simulink model "Ecotron"  (R2019b)
settings: Solver=FixedStepAuto  StartTime=0.0  StopTime=1  FixedStep=0.001  RelTol=1e-3  EnableMultiTasking=on
InitFcn:
  | EcoCoder_PreCheckLic();
libraries: CoderSF_BSW_Libs x228, SF_CanService_Libs x49, simulink x33, dspstat3 x6
(part 1 of 6)
settings Model: Param_HCUVersion=EH2275A02  Creator=btunc  LastModifiedBy=bayra
settings SolverCC: AutoInsertRateTranBlk=on
settings DataIOCC: SaveFormat=Structure  SignalLoggingSaveFormat=ModelDataLogs  SaveOutput=off  SignalLogging=off  DSMLogging=off  SaveTime=off  ReturnWorkspaceOutputs=off
settings OptimizationCC: DefaultParameterBehavior=Inlined  InlineInvariantSignals=on  EnhancedBackFolding=on  StrengthReduction=on  EnableMemcpy=off  PassReuseOutputArgsAs=Individual arguments  EfficientFloat2IntCast=on  LifeSpan=1  SimCompilerOptimization=on  OptimizeBlockOrder=speed  DifferentSizesBufferReuse=on  EfficientTunableParamExpr=on
settings DebuggingCC: AlgebraicLoopMsg=none  ArtificialAlgebraicLoopMsg=none  SaveWithDisabledLinksMsg=none  SaveWithParameterizedLinksMsg=none  CheckSSInitialOutputMsg=off  UnderspecifiedInitializationDetection=Classic  SignalResolutionControl=TryResolveAll  BlockPriorityViolationMsg=error  MinStepSizeMsg=none  InheritedTsInSrcMsg=none  MultiTaskDSMMsg=none  MultiTaskCondExecSysMsg=none  MultiTaskRateTransMsg=warning  TasksWithSamePriorityMsg=none  SigSpecEnsureSampleTimeMsg=none  IntegerOverflowMsg=error  Int32ToFloatConvMsg=none  ParameterPrecisionLossMsg=none  ParameterTunabilityLossMsg=none  FixptConstOverflowMsg=error  FcnCallInpInsideContextMsg=warning  UnconnectedInputMsg=error  UnconnectedOutputMsg=error  UnconnectedLineMsg=error  FrameProcessingCompatibilityMsg=none  BusObjectLabelMismatch=none  RootOutportRequireBusObject=none  UnknownTsInhSupMsg=none  ModelReferenceDataLoggingMessage=none  OperatingPointInterfaceChecksumMismatchMsg=none  SFUnusedDataAndEventsDiag=none  SFUnexpectedBacktrackingDiag=none  SFInvalidInputDataAccessInChartInitDiag=none  SFNoUnconditionalDefaultTransitionDiag=none  SFTransitionOutsideNaturalParentDiag=none  SFUnreachableExecutionPathDiag=none
settings HardwareCC: ProdBitPerPointer=32  ProdBitPerSizeT=32  ProdBitPerPtrDiffT=32  ProdLargestAtomicFloat=None  ProdWordSize=32  ProdHWDeviceType=Infineon->TriCore
settings ModelReferenceCC: UpdateModelReferenceTargets=Force  ModelReferenceNumInstancesAllowed=Single  PropagateSignalLabelsOutOfModel=off
settings SFSimCC: SFSimEcho=off  SimBuildMode=sf_make_clean  MATLABDynamicMemAlloc=off
settings RTWCC: Description=Ecotrons TC27x  SystemTargetFile=EcoCoderTC27x.tlc  GenerateMakefile=off  TemplateMakefile=ert_default_tmf  RTWVerbose=off  RetainRTWFile=on  RTWCompilerOptimization=on
settings CodeAppCC: IgnoreCustomStorageClasses=off  OperatorAnnotations=on  CustomSymbolStrGlobalVar=$N$M  CustomSymbolStrType=$N$M  CustomSymbolStrFcn=$N$M  CustomSymbolStrFcnArg=$N$M  CustomSymbolStrBlkIO=$N$M  CustomSymbolStrMacro=$N$M
settings STFCustomTargetCC: TargetLangStandard=C99 (ISO)  CodeReplacementLibrary=ANSI_C  UtilityFuncGeneration=Shared location  MultiwordLength=256  IncludeMdlTerminateFcn=off  CombineOutputUpdateFcns=on  SuppressErrorStatus=on  ERTCustomFileBanners=on  SupportNonFinite=off  SupportComplex=off  SupportContinuousTime=off  SupportNonInlinedSFcns=off  MATLABClassNameForMDSCustomization=Simulink.SoftwareTarget.ERTCustomization  SystemTargetFile=EcoCoderTC27x.tlc
settings ERTTargetCC: TargetLangStandard=C99 (ISO)  CodeReplacementLibrary=ANSI_C  UtilityFuncGeneration=Shared location  ParMdlRefBuildCompliant=off  CompOptLevelCompliant=off  ConcurrentExecutionCompliant=off  IncludeMdlTerminateFcn=off  SuppressErrorStatus=on  SupportNonFinite=off  SupportComplex=off  RemoveResetFunc=off  ModelStepFunctionPrototypeControlCompliant=off  CPPClassGenCompliant=off  UseToolchainInfoCompliant=off  GenerateASAP2=on  InlinedParameterPlacement=NonHierarchical  ERTCustomFileTemplate=MPC5644A_file_process.tlc  ERTFilePackagingFormat=Compact  PreserveIfCondition=on  ConvertIfToSwitch=off  PreserveExternInFcnDecls=off  SuppressUnreachableDefaultCases=off

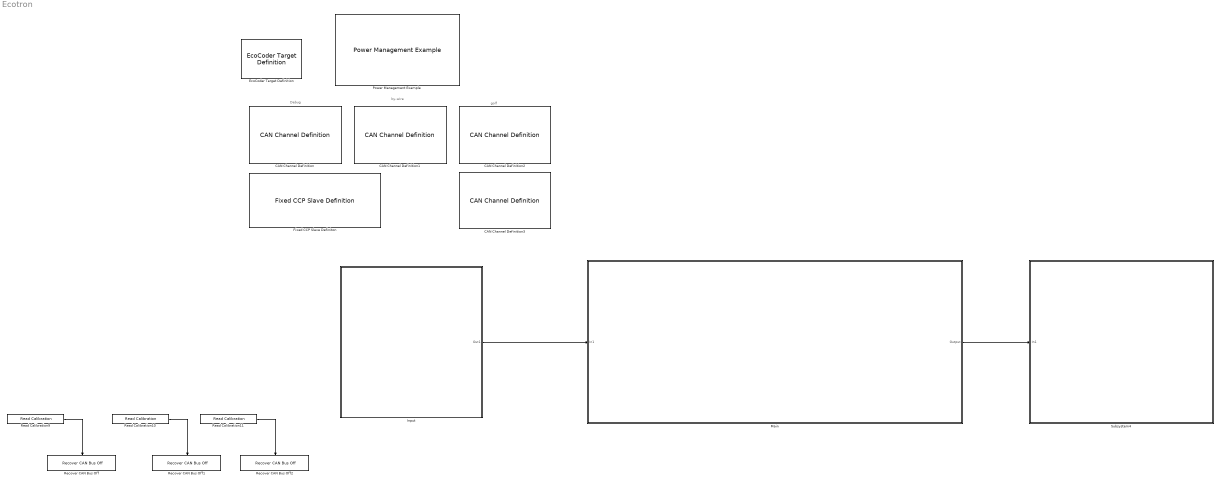
== system Ecotron ==
  note: golf
  note: by-wire
  note: Debug
  CAN Channel Definition : CoderSF_BSW_Libs/CAN/CAN Channel Definition  channel=CAN_A  can_en=on  can_idfilter=off  can_rxextended=off  can_rxMask=hex2dec('7ff')  can_rxID=hex2dec('100')  can_baudrateIndex=500  can_txbuffer_size=100  can_rxbuffer_size=1  can_en_fd=off  nominalSamplePoint=7500  can_baudrateIndex_data=500  fastSamplePoint=7500  canfd_txbuffer_size=5  EcoCoderBlockID=C001_CANDef
      settings: SourceProductName=EcoCoder Blocks
  CAN Channel Definition1 : CoderSF_BSW_Libs/CAN/CAN Channel Definition  channel=CAN_C  can_en=on  can_idfilter=off  can_rxextended=off  can_rxMask=hex2dec('7ff')  can_rxID=hex2dec('100')  can_baudrateIndex=500  can_txbuffer_size=20  can_rxbuffer_size=1  can_en_fd=off  nominalSamplePoint=7500  can_baudrateIndex_data=500  fastSamplePoint=7500  canfd_txbuffer_size=5  EcoCoderBlockID=C001_CANDef
      settings: SourceProductName=EcoCoder Blocks
  CAN Channel Definition2 : CoderSF_BSW_Libs/CAN/CAN Channel Definition  channel=CAN_B  can_en=on  can_idfilter=off  can_rxextended=off  can_rxMask=0  can_rxID=hex2dec('B5')  can_baudrateIndex=500  can_txbuffer_size=20  can_rxbuffer_size=1  can_en_fd=off  nominalSamplePoint=7500  can_baudrateIndex_data=500  fastSamplePoint=7500  canfd_txbuffer_size=5  EcoCoderBlockID=C001_CANDef
      settings: SourceProductName=EcoCoder Blocks
  CAN Channel Definition3 : CoderSF_BSW_Libs/CAN/CAN Channel Definition  channel=CAN_D  can_en=on  can_idfilter=off  can_rxextended=off  can_rxMask=hex2dec('7ff')  can_rxID=hex2dec('100')  can_baudrateIndex=500  can_txbuffer_size=20  can_rxbuffer_size=1  can_en_fd=off  nominalSamplePoint=7500  can_baudrateIndex_data=500  fastSamplePoint=7500  canfd_txbuffer_size=5  EcoCoderBlockID=C001_CANDef
      settings: SourceProductName=EcoCoder Blocks
  EcoCoder Target Definition : CoderSF_BSW_Libs/EcoCoder Target Definition  targetECU=EH2275A02  EcoCoderBlockID=T001_Target  enNoTriggerCall=on  flgBlockReduction=on  flgShowDebugDisp=off  flgDisTargetOutFIleCounter=off  flgClearAllOldFiles=on  tc275_cal_len=hex2dec('00008000')  ipVal='192.168.0.123'  userName='nvidia'  passWord='nvidia'  workSpace='~/cmake_ws'  libraryLink=''  enExt=on  portExt=17725  internal_flash=[hex2dec('00020000'),hex2dec('000E0000')]  cal_rom_phy=[hex2dec('00010000'),hex2dec('00002000')]  cal_ram_wp=[hex2dec('4000F000'),hex2dec('00002000')]  cal_ram_msm=[hex2dec('40000000'),hex2dec('00002000')]  var_ram_wp=[hex2dec('40002000'),hex2dec('0000D000')]  write_back_fixed_ram=[hex2dec('40011000'),hex2dec('00001000')]  write_back_unfixed_ram=[hex2dec('40012000'),hex2dec('00001000')]  stack=[hex2dec('40013000'),hex2dec('00001000')]
      settings: AttributesFormatString=Target :%<targetECU>  SourceProductName=EcoCoder Blocks
  Fixed CCP Slave Definiton : CoderSF_BSW_Libs/CCP/Fixed CCP Slave Definition  ccp_enSet=on  ccp_disASW=on  channel=CAN_A  stationaddressSet=hex2dec('0112')  croidSet=hex2dec('100')  dtoidSet=hex2dec('101')  daqidSet=[hex2dec('101') hex2dec('101') hex2dec('101') hex2dec('102')]  daqpidSet=[hex2dec('0') hex2dec('3C') hex2dec('78') hex2dec('0')]  daqlenSet=[hex2dec('0') hex2dec('20') hex2dec('30') hex2dec('30')]  daqperSet=[5 20 100 0]  EcoCoderBlockID=C002_CCP21Conf
      settings: SourceProductName=EcoCoder Blocks
  Input : Subsystem
  "Main " : Subsystem
  Power Management Example : CoderSF_BSW_Libs/System Management Blocks/Power Management Example  Priority=1  flgKeyFromIn=off  tasktimeIndex=Task_L5ms  tKeyOffDelaySet=0.5  flgResetSWEnSet=1  tDbncKeyOffFallSet=0.1  tDbncKeyOffRiseSet=0.1  facAd2VoltSet=109/27846  uKeyOffThrSet=1  uKeyOnHystSet=1  flgCANRxLiveCheckEn=0  flgEnPwrDwnFailReset=0  flgNVMEn=off  tShtDwnWait=500  flgPwrDwnByEdgeTrigger=off  EcoCoderBlockID=PME001_Def
      settings: AttributesFormatString=Priority:%<Priority>  SourceProductName=EcoCoder Blocks
  Read Calibration10 : CoderSF_BSW_Libs/Calibration & Measurement/Read Calibration  variable_name=CANB_recover  variable_value=0  variable_type=single  variable_min=[]  variable_max=[]  unitStr=""  descStr=""
      settings: AttributesFormatString=value:%<variable_value> type:%<variable_type> max:%<variable_max> Min:%<variable_min>  SourceProductName=EcoCoder Blocks
  Read Calibration11 : CoderSF_BSW_Libs/Calibration & Measurement/Read Calibration  variable_name=CANC_recover  variable_value=0  variable_type=single  variable_min=[]  variable_max=[]  unitStr=""  descStr=""
      settings: AttributesFormatString=value:%<variable_value> type:%<variable_type> max:%<variable_max> Min:%<variable_min>  SourceProductName=EcoCoder Blocks
  Read Calibration9 : CoderSF_BSW_Libs/Calibration & Measurement/Read Calibration  variable_name=CANA_recover  variable_value=0  variable_type=single  variable_min=[]  variable_max=[]  unitStr=""  descStr=""
      settings: AttributesFormatString=value:%<variable_value> type:%<variable_type> max:%<variable_max> Min:%<variable_min>  SourceProductName=EcoCoder Blocks
  Recover CAN Bus Off : CoderSF_BSW_Libs/CAN/Recover CAN Bus Off  channel=CAN_A
      settings: SourceProductName=EcoCoder Blocks
  Recover CAN Bus Off1 : CoderSF_BSW_Libs/CAN/Recover CAN Bus Off  channel=CAN_B
      settings: SourceProductName=EcoCoder Blocks
  Recover CAN Bus Off2 : CoderSF_BSW_Libs/CAN/Recover CAN Bus Off  channel=CAN_C
      settings: SourceProductName=EcoCoder Blocks
  Subsystem4 : Subsystem
  wires:
  Read Calibration9/1 -> Recover CAN Bus Off/Enable
  Read Calibration10/1 -> Recover CAN Bus Off1/Enable
  Read Calibration11/1 -> Recover CAN Bus Off2/Enable
  Input/1(Out1) -> "Main "/1(In1)
  "Main "/1(Output) -> Subsystem4/1(In1)

== system Ecotron/Input ==
  Bus Creator : BusCreator  Inputs=3
  By-wire : Subsystem
  Golf : Subsystem
  PC : Subsystem
  Out1 : Outport
  wires:
  By-wire/1(bywire) -> Bus Creator/1  "By-wire"
  Golf/1("Golf ") -> Bus Creator/2  "vehicle"
  Bus Creator/1 -> Out1/1
  PC/1(Output) -> Bus Creator/3  "PC"

== system Ecotron/Main  ==
  In1 : Inport
  Bus Creator : BusCreator  Inputs=2
  Bus Creator1 : BusCreator  Inputs=3
  Bus Creator2 : BusCreator  Inputs=5
  Err Handler : Subsystem
  Gear : Subsystem
  LateralControl : Subsystem
  "LongControl " : Subsystem
  Mode Select : Subsystem
  PDS StartupShutdown : Subsystem
  Output : Outport
  wires:
  In1/1 -> Bus Creator1/1, Bus Creator/1, Err Handler/1(In1)  "input"
  Err Handler/1(Out1) -> Bus Creator/2, Bus Creator1/3  "Errors"
  Bus Creator/1 -> Mode Select/1(In1)
  Mode Select/1(Output) -> Bus Creator1/2  "mode"
  Bus Creator1/1 -> Bus Creator2/1, LateralControl/1(In1), PDS StartupShutdown/1(In1), "LongControl "/1(In1), Gear/1(input)  "input"
  Gear/1(Output) -> Bus Creator2/2  "gearMSGTrigger"
  "LongControl "/1(Out1) -> Gear/2(longitudinal), Bus Creator2/3  "longitudinal"
  Bus Creator2/1 -> Output/1
  LateralControl/1(Out1) -> Bus Creator2/4  "Steer"
  PDS StartupShutdown/1(Out1) -> Bus Creator2/5  "PDSscript"

== system Ecotron/Subsystem4 ==
  In1 : Inport
  Brake : Subsystem
  Bus Selector : BusSelector  OutputSignals=Steer,gearMSGTrigger
  "Button cntrl " : Subsystem
  Gas : Subsystem
  Gear : Subsystem
  PC : Subsystem
  PDS : Subsystem
  "Steering Control " : Subsystem
  wires:
  Bus Selector/2 -> Gear/1(Gear_trigger)  "<gearMSGTrigger>"
  Bus Selector/1 -> "Steering Control "/1(inputBus)  "<Steer>"
  In1/1 -> Brake/1(Input), Gas/1(input), PC/1(In1), "Button cntrl "/1(Input), PDS/1(In1), Bus Selector/1

== system Ecotron/Input/By-wire ==
  Bus Creator : BusCreator  Inputs=4
  PDS : Subsystem
  Robeff Brake ECU : Subsystem
  Robeff EPAS ECU : Subsystem
  Throttle Controller : Subsystem
  bywire : Outport
  wires:
  Robeff EPAS ECU/1(EPAS) -> Bus Creator/1  "EPAS"
  Throttle Controller/1(Throttle) -> Bus Creator/3  "Throttle"
  Bus Creator/1 -> bywire/1
  PDS/1(PDS) -> Bus Creator/4  "PDS"
  Robeff Brake ECU/1(RBF_Brake) -> Bus Creator/2  "RBF_Brake"

== system Ecotron/Input/Golf ==
  BCM_01 : Subsystem
  Brake : Subsystem
  Brake and Steering Feedback Echo : Subsystem
  Bus Creator : BusCreator  Inputs=16
  EPB_01 : Subsystem
  ESP_05 : Subsystem
  Gateway_72 : Subsystem
  Getriebe_1 : Subsystem
  Getriebe_11 : Subsystem
  Getriebe_2 : Subsystem
  Kombi_02 : Subsystem
  LWl : Subsystem
  Motor_11 : Subsystem
  Motor_12 : Subsystem
  Motor_14 : Subsystem
  Motor_20 : Subsystem
  Subsystem : Subsystem
  WheelSpeed : Subsystem
  "Golf " : Outport
  wires:
  WheelSpeed/1("WheelSpeed ") -> Bus Creator/3  "WheelSpeed"
  Brake/1(Brake) -> Bus Creator/2  "BrakePedal"
  LWl/1(LWI) -> Bus Creator/1  "LWI"
  Bus Creator/1 -> "Golf "/1
  EPB_01/1(Acceleration) -> Bus Creator/6  "Acceleration"
  Motor_20/1(Accelerator_Pedal) -> Bus Creator/7  "Acc_Pedal_POS"
  Motor_14/1(KL75) -> Bus Creator/8  "Kontak"
  Gateway_72/1(Signal) -> Bus Creator/9  "Signal"
  Motor_12/1(MatorRPM) -> Bus Creator/5  "MotorRotationSpeed"
  Subsystem/1(GearSwitch) -> Bus Creator/4  "gear"
  BCM_01/1(HazardLight) -> Bus Creator/10  "Hazard"
  Kombi_02/1(Fuel_Tank) -> Bus Creator/11  "Fuel"
  Motor_11/1(MatorTorque) -> Bus Creator/12  "MotorTorque"
  Getriebe_11/1(GearLevel) -> Bus Creator/13  "GearLevel"
  Getriebe_1/1(ACC) -> Bus Creator/14  "ACC"
  Getriebe_2/1(TSK) -> Bus Creator/15  "TSK"
  ESP_05/1(ESP_05) -> Bus Creator/16  "BrakePressure"

== system Ecotron/Input/PC ==
  Bus Creator : BusCreator  Inputs=4
  FrontWheelCommands : Subsystem
  LongitudinalCommands : Subsystem
  LongitudinalCommandsV2 : Subsystem
  Vehicle_Commands : Subsystem
  Output : Outport
  wires:
  Vehicle_Commands/1(Out1) -> Bus Creator/1  "VehicleCMD"
  FrontWheelCommands/1(Out2) -> Bus Creator/2  "FrontWheelCMD"
  LongitudinalCommands/1(Out2) -> Bus Creator/3  "LongCMD"
  LongitudinalCommandsV2/1(Out2) -> Bus Creator/4  "LongV2CMD"
  Bus Creator/1 -> Output/1

== system Ecotron/Main /Err Handler ==
  In1 : Inport
  Bus Creator : BusCreator  Inputs=6
  Check Brake Err : Subsystem
  Check EPAS Err : Subsystem
  Check PDS Errors : Subsystem
  Check Throttle ECU Errors : Subsystem
  MotorStatus : Subsystem
  Subsystem : Subsystem
  Out1 : Outport
  wires:
  Check Brake Err/1(Out1) -> Bus Creator/5  "Brake_Err"
  In1/1 -> Subsystem/1(In1), Check Brake Err/1(In1), Check EPAS Err/1(In1), MotorStatus/1(In1), Check PDS Errors/1(In1), Check Throttle ECU Errors/1(In1)
  MotorStatus/1(Motor) -> Bus Creator/1  "Motor"
  Check PDS Errors/1(Out1) -> Bus Creator/2  "PDS_Err"
  Check Throttle ECU Errors/1(Out1) -> Bus Creator/3  "Throttle_ECU_Err"
  Bus Creator/1 -> Out1/1
  Check EPAS Err/1(Epas_Errors) -> Bus Creator/4  "Epas_Err"
  Subsystem/1(Out1) -> Bus Creator/6  "PC_HeartBeatErr"

== system Ecotron/Main /Gear ==
  input : Inport
  longitudinal : Inport  Port=2
  " Override Probe" : CoderSF_BSW_Libs/Calibration & Measurement/ Override Probe  variableName=Set_GearEnable  variableValue=1  overrideValue=0  variableDataType=single  variableMin=[]  variableMax=[]  variableUnitStr=""  variableDescStr=""
      settings: SourceProductName=EcoCoder Blocks
  Bus Selector : BusSelector  OutputSignals=input.vehicle.gear.GOLF_CurrentGear,input.vehicle.gear.Msg.Available,input.vehicle.Acceleration.GOLF_HandBrakeStatus,input.PC.VehicleCMD.PC_gear,mode
  Bus Selector1 : BusSelector  OutputSignals=stopMode
  Compare To Constant : simulink/Logic and Bit Operations/Compare To Constant  relop===  const=1  OutDataTypeStr=boolean
  Constant : Constant  OutDataTypeStr=uint8
  Gear_Control : Subsystem
  Switch : Switch  Criteria=u2 > Threshold  Threshold=0.5
  Output : Outport
  wires:
  Bus Selector/2 -> Gear_Control/2(Available)  "<Available>"
  Bus Selector/1 -> Gear_Control/1(GOLF_CurrentGear)  "<GOLF_CurrentGear>"
  input/1 -> Bus Selector/1
  " Override Probe"/1 -> Gear_Control/4(Enable)  "Set_GearEnableOvrMsr"
  Gear_Control/1(Gear_Trigger) -> Output/1
  Bus Selector/3 -> Switch/2  "<GOLF_HandBrakeStatus>"
  Constant/1 -> Switch/1
  Switch/1 -> Gear_Control/3("Set_gear ")
  Bus Selector/4 -> Switch/3  "<PC_gear>"
  Bus Selector/5 -> " Override Probe"/1  "<mode>"
  longitudinal/1 -> Bus Selector1/1
  Bus Selector1/1 -> Compare To Constant/1  "<stopMode>"
  Compare To Constant/1 -> Gear_Control/5(ParkEnable)

== system Ecotron/Main /LateralControl ==
  In1 : Inport
  Bus Creator : BusCreator  Inputs=4
  Bus Selector : BusSelector  OutputSignals=mode,input.vehicle.WheelSpeed.GOLF_BRWheelSpeed,input.By-wire.EPAS.EPAS_Msg3.EPAS_DriverIntervention_overrideOvrMsr,input.PC.FrontWheelCMD.PC_SetFrontWheelAngle
  Chart : Stateflow chart  BlockKeywords=__PRM__SERIALIZED__DATA__:Stateflow Chart,Stateflow Diagram  TreatAsAtomicUnit=on
  Read Calibration : CoderSF_BSW_Libs/Calibration & Measurement/Read Calibration  variable_name=EPAS_MaxSpeed  variable_value=360  variable_type=single  variable_min=[]  variable_max=[]  unitStr=""  descStr=""
      settings: AttributesFormatString=value:%<variable_value> type:%<variable_type> max:%<variable_max> Min:%<variable_min>  SourceProductName=EcoCoder Blocks
  Steering Map : Subsystem
  Write and Read Measurement : CoderSF_BSW_Libs/Calibration & Measurement/Write and Read Measurement  variable_name=debug_EPASmode  variable_value=0  variable_type=uint8  numD=1  unitStr=""  descStr=""
      settings: AttributesFormatString=type:%<variable_type> Dimensions:%<numD>  SourceProductName=EcoCoder Blocks
  Write and Read Measurement1 : CoderSF_BSW_Libs/Calibration & Measurement/Write and Read Measurement  variable_name=debug_EPASsetsteer  variable_value=0  variable_type=single  numD=1  unitStr=""  descStr=""
      settings: AttributesFormatString=type:%<variable_type> Dimensions:%<numD>  SourceProductName=EcoCoder Blocks
  Write and Read Measurement2 : CoderSF_BSW_Libs/Calibration & Measurement/Write and Read Measurement  variable_name=debug_EPASspeedlimit  variable_value=0  variable_type=single  numD=1  unitStr=""  descStr=""
      settings: AttributesFormatString=type:%<variable_type> Dimensions:%<numD>  SourceProductName=EcoCoder Blocks
  Write and Read Measurement3 : CoderSF_BSW_Libs/Calibration & Measurement/Write and Read Measurement  variable_name=debug_EPAS_ECU_reset  variable_value=0  variable_type=boolean  numD=1  unitStr=""  descStr=""
      settings: AttributesFormatString=type:%<variable_type> Dimensions:%<numD>  SourceProductName=EcoCoder Blocks
  Out1 : Outport
  wires:
  In1/1 -> Bus Selector/1
  Bus Selector/1 -> Chart/1(AutonomyEnable)  "<mode>"
  Bus Creator/1 -> Out1/1
  Write and Read Measurement/1 -> Bus Creator/1  "debug_EPASmode"
  Write and Read Measurement1/1 -> Bus Creator/2  "debug_EPASsetsteer"
  Write and Read Measurement2/1 -> Bus Creator/3  "debug_EPASspeedlimit"
  Chart/1(EPAS_mode) -> Write and Read Measurement/1
  Chart/2(EPAS_SteeringPosCMD) -> Write and Read Measurement1/1
  Chart/3(EPAS_Speedlimit) -> Write and Read Measurement2/1
  Chart/4(Epas_ECU_reset) -> Write and Read Measurement3/1
  Write and Read Measurement3/1 -> Bus Creator/4  "debug_EPAS_ECU_reset"
  Bus Selector/4 -> Steering Map/1(Wheel Rad)  "<PC_SetFrontWheelAngle>"
  Read Calibration/1 -> Chart/4(MaxEPASSpeed)
  Bus Selector/2 -> Chart/2(Vehicle_Speed)  "<GOLF_BRWheelSpeed>"
  Bus Selector/3 -> Chart/3(EPAS_intervention)  "<EPAS_DriverIntervention_overrideOvrMsr>"
  Steering Map/1(Steering Wheel Degree) -> Chart/5(Set_SteeringPos)

== system Ecotron/Main /LongControl  ==
  In1 : Inport
  ACC Control : Subsystem
  Brake Calib logic : Subsystem
  Bus Creator : BusCreator  Inputs=4
  Bus Selector : BusSelector  OutputSignals=mode,input.PC.VehicleCMD.PC_LongMode,input.PC.LongV2CMD.PC_SetBrakePos,input.PC.LongV2CMD.PC_SetGasPos
  Chart : Stateflow chart  Commented=on  BlockKeywords=__PRM__SERIALIZED__DATA__:Stateflow Chart,Stateflow Diagram  TreatAsAtomicUnit=on
  Out1 : Outport
  wires:
  Bus Selector/1 -> Chart/1(AutonomyEnable)  "<mode>"
  Bus Selector/2 -> Chart/2(LongMode)  "<PC_LongMode>"
  Bus Selector/3 -> Chart/3(PC_Brake)  "<PC_SetBrakePos>"
  Bus Selector/4 -> Chart/4(PC_Throttle)  "<PC_SetGasPos>"
  Bus Creator/1 -> Out1/1
  In1/1 -> Brake Calib logic/1(In1), ACC Control/1(In2), Bus Selector/1
  Brake Calib logic/1(Out1) -> Bus Creator/3  "BrakeCalibCMD"
  ACC Control/1(gas) -> Bus Creator/2  "Throttle_out"
  ACC Control/2(brake) -> Bus Creator/1  "Brake_out"
  ACC Control/3(StopMode) -> Bus Creator/4  "stopMode"

== system Ecotron/Main /Mode Select ==
  In1 : Inport
  " Override Probe" : CoderSF_BSW_Libs/Calibration & Measurement/ Override Probe  variableName=debug_otonomEnable  variableValue=0  overrideValue=0  variableDataType=boolean  variableMin=[]  variableMax=[]  variableUnitStr=""  variableDescStr=""
      settings: SourceProductName=EcoCoder Blocks
  " Override Probe1" : CoderSF_BSW_Libs/Calibration & Measurement/ Override Probe  variableName=debug_otonomDisable  variableValue=0  overrideValue=0  variableDataType=boolean  variableMin=[]  variableMax=[]  variableUnitStr=""  variableDescStr=""
      settings: SourceProductName=EcoCoder Blocks
  " Override Probe2" : CoderSF_BSW_Libs/Calibration & Measurement/ Override Probe  variableName=debug_PCheardbeat  variableValue=0  overrideValue=0  variableDataType=boolean  variableMin=[]  variableMax=[]  variableUnitStr=""  variableDescStr=""
      settings: SourceProductName=EcoCoder Blocks
  Bus Selector1 : BusSelector  OutputSignals=Errors.Motor.isMotorRunning,Errors.Motor.Kl75,Errors.PDS_Err.PDS_HeartbeatErr,Errors.PDS_Err.PDS_BUSErr,Errors.PDS_Err.By-wirePowerErr,Errors.PDS_Err.EPASPowerErr,Errors.PDS_Err.BrakePowerErr,Errors.Throttle_ECU_Err.GasPedalintervention,Errors.Epas_Err.EPAS_SystemErr,Errors.Brake_Err.Brake_SystemErr,input.By-wire.EPAS.EPAS_Msg3.EPAS_DriverIntervention_overrideOvrMsr,input.By-wire.RBF_Brake.EPAS_Msg3.BBW_DriverIntervention,Errors.Brake_Err.Brake_HeartBeatErr,Errors.Epas_Err.EPAS_HeartbeatErr,Errors.PC_HeartBeatErr
  Bus Selector2 : BusSelector  OutputSignals=input.PC.VehicleCMD.PC_mode,input.vehicle.Acceleration.GOLF_HandBrakeStatus
  Chart : Stateflow chart  BlockKeywords=__PRM__SERIALIZED__DATA__:Stateflow Chart,Stateflow Diagram  TreatAsAtomicUnit=on
  Compare To Constant : simulink/Logic and Bit Operations/Compare To Constant  relop===  const=1  OutDataTypeStr=boolean
  Compare To Constant1 : simulink/Logic and Bit Operations/Compare To Constant  relop=~=  const=1  OutDataTypeStr=boolean
  NOT : Logic  Operator=NOT  IconShape=distinctive  AllPortsSameDT=off  OutDataTypeStr=boolean
  NOT1 : Logic  Operator=NOT  IconShape=distinctive  AllPortsSameDT=off  OutDataTypeStr=boolean
  OR : Logic  Operator=OR  Inputs=15  IconShape=distinctive  AllPortsSameDT=off  OutDataTypeStr=boolean
  Rising Edge1 : CoderSF_BSW_Libs/Application Base Blocks/Rising Edge  InitialCondition=off
      settings: SourceProductName=EcoCoder Blocks
  Rising Edge2 : CoderSF_BSW_Libs/Application Base Blocks/Rising Edge  InitialCondition=off
      settings: SourceProductName=EcoCoder Blocks
  Rising Edge3 : CoderSF_BSW_Libs/Application Base Blocks/Rising Edge  InitialCondition=off
      settings: SourceProductName=EcoCoder Blocks
  Write Measurement : CoderSF_BSW_Libs/Calibration & Measurement/Write Measurement  variable_name=debug_Mode  variable_value=0  variable_type=boolean  numD=1  unitStr=""  descStr=""
      settings: AttributesFormatString=type:%<variable_type> Dimensions:%<numD>  SourceProductName=EcoCoder Blocks
  Write Measurement3 : CoderSF_BSW_Libs/Calibration & Measurement/Write Measurement  variable_name=debug_Errors  variable_value=0  variable_type=boolean  numD=1  unitStr=""  descStr=""
      settings: AttributesFormatString=type:%<variable_type> Dimensions:%<numD>  SourceProductName=EcoCoder Blocks
  Output : Outport
  wires:
  In1/1 -> Bus Selector1/1, Bus Selector2/1
  Bus Selector1/1 -> NOT/1  "<isMotorRunning>"
  Bus Selector1/2 -> NOT1/1  "<Kl75>"
  Bus Selector1/3 -> OR/3  "<PDS_HeartbeatErr>"
  Bus Selector1/4 -> OR/4  "<PDS_BUSErr>"
  Bus Selector1/5 -> OR/5  "<By-wirePowerErr>"
  Bus Selector1/6 -> OR/6  "<EPASPowerErr>"
  Bus Selector1/7 -> OR/7  "<BrakePowerErr>"
  Bus Selector1/8 -> OR/8  "<GasPedalintervention>"
  Bus Selector1/9 -> OR/9  "<EPAS_SystemErr>"
  Bus Selector1/10 -> OR/10  "<Brake_SystemErr>"
  OR/1 -> Chart/1(Errors), Write Measurement3/1
  " Override Probe"/1 -> Chart/2(AutonomyEnable)  "debug_otonomEnableOvrMsr"
  Chart/1(Mode) -> Output/1, Write Measurement/1  "autonomy_Enable"
  NOT/1 -> OR/1
  NOT1/1 -> OR/2
  Bus Selector1/11 -> Rising Edge2/1  "<EPAS_DriverIntervention_overrideOvrMsr>"
  Bus Selector1/12 -> Rising Edge1/1  "<BBW_DriverIntervention>"
  Bus Selector1/13 -> OR/13  "<Brake_HeartBeatErr>"
  Bus Selector1/14 -> OR/14  "<EPAS_HeartbeatErr>"
  Bus Selector2/1 -> Compare To Constant1/1, Compare To Constant/1  "<PC_mode>"
  Rising Edge1/1 -> OR/12
  Rising Edge2/1 -> OR/11
  Compare To Constant/1 -> Rising Edge3/1
  Bus Selector1/15 -> " Override Probe2"/1  "<PC_HeartBeatErr>"
  Rising Edge3/1 -> " Override Probe"/1
  Compare To Constant1/1 -> " Override Probe1"/1
  " Override Probe1"/1 -> Chart/3(AutonomyDisable)  "debug_otonomDisableOvrMsr"
  Bus Selector2/2 -> Chart/4(HandBrake)  "<GOLF_HandBrakeStatus>"
  " Override Probe2"/1 -> OR/15  "debug_PCheardbeatOvrMsr"

== system Ecotron/Main /PDS StartupShutdown ==
  In1 : Inport
  Bus Creator : BusCreator  Inputs=3
  Bus Selector : BusSelector  OutputSignals=input.By-wire.PDS.Status.PDS_Status1
  Chart : Stateflow chart  BlockKeywords=__PRM__SERIALIZED__DATA__:Stateflow Chart,Stateflow Diagram  TreatAsAtomicUnit=on
  Compare To Constant : simulink/Logic and Bit Operations/Compare To Constant  relop=>  const=0  OutDataTypeStr=boolean
  Falling Edge : CoderSF_BSW_Libs/Application Base Blocks/Falling Edge  InitialCondition=off
      settings: SourceProductName=EcoCoder Blocks
  Rising Edge : CoderSF_BSW_Libs/Application Base Blocks/Rising Edge  InitialCondition=on
      settings: SourceProductName=EcoCoder Blocks
  Out1 : Outport
  wires:
  In1/1 -> Bus Selector/1
  Bus Selector/1 -> Compare To Constant/1  "<PDS_Status1>"
  Compare To Constant/1 -> Falling Edge/1, Rising Edge/1
  Rising Edge/1 -> Chart/1(risingedge)
  Falling Edge/1 -> Chart/2(fallingedge)
  Chart/1(Channel) -> Bus Creator/1
  Chart/2(Onoff) -> Bus Creator/2
  Chart/3(Msgtrigger) -> Bus Creator/3
  Bus Creator/1 -> Out1/1

== system Ecotron/Subsystem4/Brake ==
  Input : Inport
  " Override Probe" : CoderSF_BSW_Libs/Calibration & Measurement/ Override Probe  variableName=Set_Brake_Pos  variableValue=0  overrideValue=0  variableDataType=single  variableMin=[]  variableMax=[]  variableUnitStr=""  variableDescStr=""
      settings: SourceProductName=EcoCoder Blocks
  " Override Probe1" : CoderSF_BSW_Libs/Calibration & Measurement/ Override Probe  variableName=Brake_Reset  variableValue=0  overrideValue=0  variableDataType=uint8  variableMin=[]  variableMax=[]  variableUnitStr=""  variableDescStr=""
      settings: SourceProductName=EcoCoder Blocks
  Bus Selector : BusSelector  OutputSignals=longitudinal.Brake_out,input.mode,Steer.debug_EPAS_ECU_reset,longitudinal.BrakeCalibCMD
  Constant6 : Constant  Value=0
  Read Calibration1 : CoderSF_BSW_Libs/Calibration & Measurement/Read Calibration  variable_name=Brake_ControlMode  variable_value=0  variable_type=single  variable_min=[]  variable_max=[]  unitStr=""  descStr=""
      settings: AttributesFormatString=value:%<variable_value> type:%<variable_type> max:%<variable_max> Min:%<variable_min>  SourceProductName=EcoCoder Blocks
  Read Calibration19 : CoderSF_BSW_Libs/Calibration & Measurement/Read Calibration  variable_name=Brake_SetDuty  variable_value=0  variable_type=uint8  variable_min=[]  variable_max=[]  unitStr=""  descStr=""
      settings: AttributesFormatString=value:%<variable_value> type:%<variable_type> max:%<variable_max> Min:%<variable_min>  SourceProductName=EcoCoder Blocks
  Send CAN Message 2 : SF_CanService_Libs/Send CAN Message   typeCAN=Connected  channel=CAN_C  mEn=off  msgInfo=RBF_DBW40_brake  msgItermStore=CommandMessage  msgIterm=CommandMessage  motoBit=off  flgNoFixed=on  tSample=Task_L10ms  modeCode=Parameterless  modeRound=Zero
  Switch2 : Switch  Criteria=u2 > Threshold  OutDataTypeStr=single
  wires:
  Read Calibration19/1 -> Send CAN Message 2/2
  " Override Probe1"/1 -> Send CAN Message 2/4  "Brake_ResetOvrMsr"
  " Override Probe"/1 -> Send CAN Message 2/3  "Set_Brake_PosOvrMsr"
  Input/1 -> Bus Selector/1
  Constant6/1 -> Switch2/3
  Switch2/1 -> " Override Probe"/1
  Bus Selector/2 -> Switch2/2  "<mode>"
  Bus Selector/1 -> Switch2/1  "<Brake_out>"
  Read Calibration1/1 -> Send CAN Message 2/1  "Brake_ControlModeOvrMsr"
  Bus Selector/3 -> " Override Probe1"/1  "<debug_EPAS_ECU_reset>"
  Bus Selector/4 -> Send CAN Message 2/5  "<BrakeCalibCMD>"

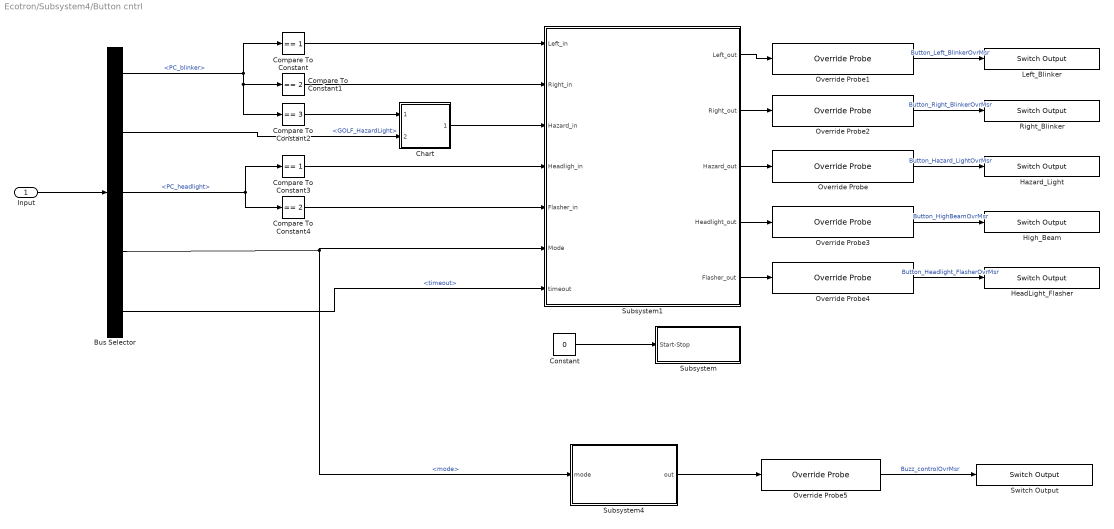
== system Ecotron/Subsystem4/Button cntrl  ==
  Input : Inport
  " Override Probe" : CoderSF_BSW_Libs/Calibration & Measurement/ Override Probe  variableName=Button_Hazard_Light  variableValue=0  overrideValue=0  variableDataType=boolean  variableMin=[]  variableMax=[]  variableUnitStr=""  variableDescStr=""
      settings: SourceProductName=EcoCoder Blocks
  " Override Probe1" : CoderSF_BSW_Libs/Calibration & Measurement/ Override Probe  variableName=Button_Left_Blinker  variableValue=0  overrideValue=0  variableDataType=boolean  variableMin=[]  variableMax=[]  variableUnitStr=""  variableDescStr=""
      settings: SourceProductName=EcoCoder Blocks
  " Override Probe2" : CoderSF_BSW_Libs/Calibration & Measurement/ Override Probe  variableName=Button_Right_Blinker  variableValue=0  overrideValue=0  variableDataType=boolean  variableMin=[]  variableMax=[]  variableUnitStr=""  variableDescStr=""
      settings: SourceProductName=EcoCoder Blocks
  " Override Probe3" : CoderSF_BSW_Libs/Calibration & Measurement/ Override Probe  variableName=Button_HighBeam  variableValue=0  overrideValue=0  variableDataType=boolean  variableMin=[]  variableMax=[]  variableUnitStr=""  variableDescStr=""
      settings: SourceProductName=EcoCoder Blocks
  " Override Probe4" : CoderSF_BSW_Libs/Calibration & Measurement/ Override Probe  variableName=Button_Headlight_Flasher  variableValue=0  overrideValue=0  variableDataType=boolean  variableMin=[]  variableMax=[]  variableUnitStr=""  variableDescStr=""
      settings: SourceProductName=EcoCoder Blocks
  " Override Probe5" : CoderSF_BSW_Libs/Calibration & Measurement/ Override Probe  variableName=Buzz_control  variableValue=0  overrideValue=0  variableDataType=boolean  variableMin=[]  variableMax=[]  variableUnitStr=""  variableDescStr=""
      settings: SourceProductName=EcoCoder Blocks
  Bus Selector : BusSelector  OutputSignals=input.input.PC.VehicleCMD.PC_blinker,input.input.vehicle.Hazard.GOLF_HazardLight,input.input.PC.VehicleCMD.PC_headlight,input.mode,input.input.PC.VehicleCMD.Msg.timeout
  Chart : Stateflow chart  BlockKeywords=__PRM__SERIALIZED__DATA__:Stateflow Chart,Stateflow Diagram  TreatAsAtomicUnit=on
  Compare To Constant : simulink/Logic and Bit Operations/Compare To Constant  relop===  const=1  OutDataTypeStr=boolean
  Compare To Constant1 : simulink/Logic and Bit Operations/Compare To Constant  relop===  const=2  OutDataTypeStr=boolean
  Compare To Constant2 : simulink/Logic and Bit Operations/Compare To Constant  relop===  const=3  OutDataTypeStr=boolean
  Compare To Constant3 : simulink/Logic and Bit Operations/Compare To Constant  relop===  const=1  OutDataTypeStr=boolean
  Compare To Constant4 : simulink/Logic and Bit Operations/Compare To Constant  relop===  const=2  OutDataTypeStr=boolean
  Constant : Constant  Value=0  OutDataTypeStr=boolean
  Hazard_Light : CoderSF_BSW_Libs/Digital I//O/Switch Output  channel=HSO08
      settings: SourceProductName=EcoCoder Blocks
  HeadLight_Flasher : CoderSF_BSW_Libs/Digital I//O/Switch Output  channel=HSO06
      settings: SourceProductName=EcoCoder Blocks
  High_Beam : CoderSF_BSW_Libs/Digital I//O/Switch Output  channel=HSO05
      settings: SourceProductName=EcoCoder Blocks
  Left_Blinker : CoderSF_BSW_Libs/Digital I//O/Switch Output  channel=HSO03
      settings: SourceProductName=EcoCoder Blocks
  Right_Blinker : CoderSF_BSW_Libs/Digital I//O/Switch Output  channel=HSO04
      settings: SourceProductName=EcoCoder Blocks
  Subsystem : Subsystem
  Subsystem1 : Subsystem
  Subsystem4 : Subsystem
  Switch Output : CoderSF_BSW_Libs/Digital I//O/Switch Output  channel=LSO23
      settings: SourceProductName=EcoCoder Blocks
  wires:
  " Override Probe1"/1 -> Left_Blinker/1  "Button_Left_BlinkerOvrMsr"
  " Override Probe"/1 -> Hazard_Light/1  "Button_Hazard_LightOvrMsr"
  " Override Probe3"/1 -> High_Beam/1  "Button_HighBeamOvrMsr"
  " Override Probe2"/1 -> Right_Blinker/1  "Button_Right_BlinkerOvrMsr"
  Input/1 -> Bus Selector/1
  " Override Probe4"/1 -> HeadLight_Flasher/1  "Button_Headlight_FlasherOvrMsr"
  Bus Selector/1 -> Compare To Constant2/1, Compare To Constant1/1, Compare To Constant/1  "<PC_blinker>"
  Compare To Constant/1 -> Subsystem1/1(Left_in)
  Compare To Constant1/1 -> Subsystem1/2(Right_in)
  Compare To Constant2/1 -> Chart/1(SetHazard)
  Bus Selector/3 -> Compare To Constant4/1, Compare To Constant3/1  "<PC_headlight>"
  Compare To Constant3/1 -> Subsystem1/4(Headligh_in)
  Compare To Constant4/1 -> Subsystem1/5(Flasher_in)
  Constant/1 -> Subsystem/1("Start-Stop ")
  Bus Selector/2 -> Chart/2(HazardState)  "<GOLF_HazardLight>"
  Chart/1(Output) -> Subsystem1/3(Hazard_in)
  Bus Selector/4 -> Subsystem4/1(mode), Subsystem1/6(Mode)  "<mode>"
  Bus Selector/5 -> Subsystem1/7(timeout)  "<timeout>"
  Subsystem1/1(Left_out) -> " Override Probe1"/1
  Subsystem1/2(Right_out) -> " Override Probe2"/1
  Subsystem1/3(Hazard_out) -> " Override Probe"/1
  Subsystem1/4(Headlight_out) -> " Override Probe3"/1
  Subsystem1/5(Flasher_out) -> " Override Probe4"/1
  " Override Probe5"/1 -> Switch Output/1  "Buzz_controlOvrMsr"
  Subsystem4/1(out) -> " Override Probe5"/1

== system Ecotron/Subsystem4/Gas ==
  input : Inport
  " Override Probe" : CoderSF_BSW_Libs/Calibration & Measurement/ Override Probe  variableName=Set_Gas  variableValue=0  overrideValue=0  variableDataType=single  variableMin=[]  variableMax=[]  variableUnitStr=""  variableDescStr=""
      settings: SourceProductName=EcoCoder Blocks
  " Override Probe1" : CoderSF_BSW_Libs/Calibration & Measurement/ Override Probe  variableName=Activate_ThrottleController  variableValue=0  overrideValue=0  variableDataType=single  variableMin=[]  variableMax=[]  variableUnitStr=""  variableDescStr=""
      settings: SourceProductName=EcoCoder Blocks
  1-D Lookup Table : Lookup_n-D  NumberOfTableDimensions=1  BreakpointsForDimension1=[0 1.6 2.4 4 5.6 6.8 8 12.4 18.8 26 32.4 39 46 53.2 59.6 66.8 73.6 80.4 87.2 94 100]  Table=[0 7 8 9 10 11 12 15 20 25 30 35 40 45 50 55 60 65 70 75 80]  InternalRulePriority=Speed  RndMeth=Simplest  InputSameDT=on
  Bus Selector1 : BusSelector  OutputSignals=longitudinal.Throttle_out,input.mode
  Send CAN Message 1 : SF_CanService_Libs/Send CAN Message   typeCAN=Connected  channel=CAN_C  mEn=off  msgInfo=Leo_accpedal  msgItermStore=Acc_Pedal_Command  msgIterm=Acc_Pedal_Command  motoBit=off  flgNoFixed=on  tSample=Task_L10ms  modeCode=Parameterless  modeRound=Zero
  wires:
  " Override Probe1"/1 -> Send CAN Message 1/2  "Activate_ThrottleControllerOvrMsr"
  Bus Selector1/1 -> 1-D Lookup Table/1  "<Throttle_out>"
  " Override Probe"/1 -> Send CAN Message 1/1  "Set_GasOvrMsr"
  input/1 -> Bus Selector1/1
  Bus Selector1/2 -> " Override Probe1"/1  "<mode>"
  1-D Lookup Table/1 -> " Override Probe"/1

== system Ecotron/Subsystem4/Gear ==
  Gear_trigger : Inport
  Bus Selector : BusSelector  OutputSignals=PtoD,NtoD,DtoN,NtoR,RtoN,PtoN,Parktrigger
  "Drive " : Subsystem
  Neutral : Subsystem
  Reverse : Subsystem
  Reverse1 : Subsystem
  Reverse2 : Subsystem
  Reverse3 : Subsystem
  Switch Output : CoderSF_BSW_Libs/Digital I//O/Switch Output  channel=HSO07
      settings: SourceProductName=EcoCoder Blocks
  wires:
  Bus Selector/3 -> Reverse/Trigger  "<DtoN>"
  Gear_trigger/1 -> Bus Selector/1
  Bus Selector/1 -> "Drive "/Enable  "<PtoD>"
  Bus Selector/2 -> Neutral/Enable  "<NtoD>"
  Bus Selector/5 -> Reverse2/Trigger  "<RtoN>"
  Bus Selector/6 -> Reverse3/Trigger  "<PtoN>"
  Bus Selector/4 -> Reverse1/Trigger  "<NtoR>"
  Bus Selector/7 -> Switch Output/1  "<Parktrigger>"

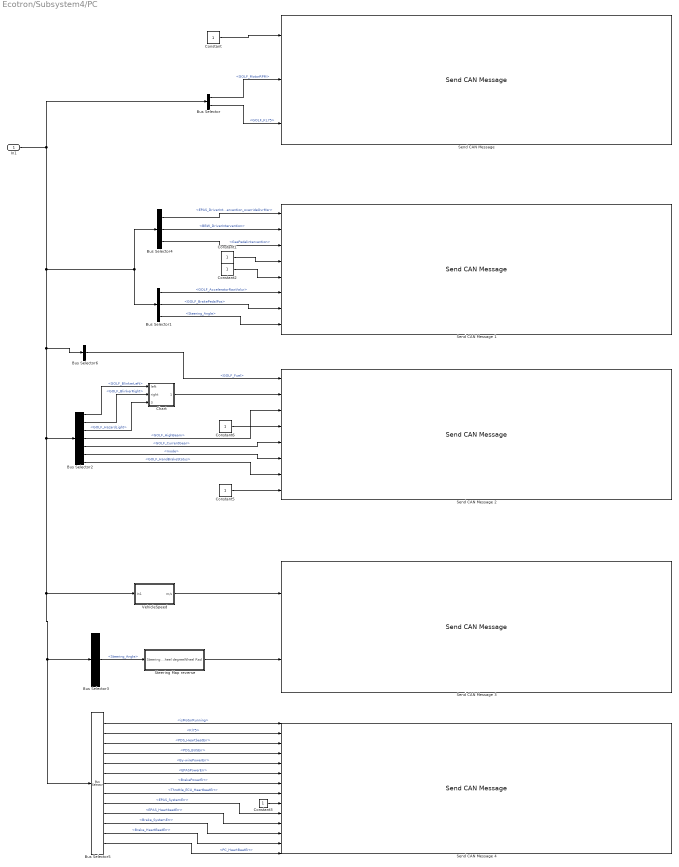
== system Ecotron/Subsystem4/PC ==
  In1 : Inport
  Bus Selector : BusSelector  OutputSignals=input.input.vehicle.MotorRotationSpeed.GOLF_MotorRPM,input.input.vehicle.Kontak.GOLF_KL75
  Bus Selector1 : BusSelector  OutputSignals=input.input.vehicle.Acc_Pedal_POS.GOLF_AcceleratorRawValur,input.input.vehicle.BrakePedal.GOLF_BrakePedalPos,input.input.vehicle.LWI.Steering_Angle
  Bus Selector2 : BusSelector  OutputSignals=input.input.vehicle.Signal.GOLF_BlinkerLeft,input.input.vehicle.Signal.GOLF_BlinkerRight,input.input.vehicle.Hazard.GOLF_HazardLight,input.input.vehicle.Signal.GOLF_HighBeam,input.input.vehicle.gear.GOLF_CurrentGear,input.mode,input.input.vehicle.Acceleration.GOLF_HandBrakeStatus
  Bus Selector3 : BusSelector  OutputSignals=input.input.vehicle.LWI.Steering_Angle
  Bus Selector4 : BusSelector  OutputSignals=input.input.By-wire.EPAS.EPAS_Msg3.EPAS_DriverIntervention_overrideOvrMsr,input.input.By-wire.RBF_Brake.EPAS_Msg3.BBW_DriverIntervention,input.Errors.Throttle_ECU_Err.GasPedalintervention
  Bus Selector5 : BusSelector  OutputSignals=input.Errors.Motor.isMotorRunning,input.Errors.Motor.Kl75,input.Errors.PDS_Err.PDS_HeartbeatErr,input.Errors.PDS_Err.PDS_BUSErr,input.Errors.PDS_Err.By-wirePowerErr,input.Errors.PDS_Err.EPASPowerErr,input.Errors.PDS_Err.BrakePowerErr,input.Errors.Throttle_ECU_Err.Throttle_ECU_HeartbeatErr,input.Errors.Epas_Err.EPAS_SystemErr,input.Errors.Epas_Err.EPAS_HeartbeatErr,input.Errors.Brake_Err.Brake_SystemErr,input.Errors.Brake_Err.Brake_HeartBeatErr,input.Errors.PC_HeartBeatErr
  Bus Selector6 : BusSelector  OutputSignals=input.input.vehicle.Fuel.GOLF_Fuel
  Chart : Stateflow chart  BlockKeywords=__PRM__SERIALIZED__DATA__:Stateflow Chart,Stateflow Diagram  TreatAsAtomicUnit=on
  Constant{,1..3,5..6} (6 alike) : Constant
  "Send CAN Message " : SF_CanService_Libs/Send CAN Message   typeCAN=Connected  channel=CAN_D  mEn=off  msgInfo=LeoDrive_vw_GOLF  msgItermStore=motor_info  msgIterm=motor_info  motoBit=off  flgNoFixed=on  tSample=Task_L10ms  modeCode=Parameterless  modeRound=Zero
  Send CAN Message 1 : SF_CanService_Libs/Send CAN Message   typeCAN=Connected  channel=CAN_D  mEn=off  msgInfo=LeoDrive_vw_GOLF  msgItermStore=MotionInfo  msgIterm=MotionInfo  motoBit=off  flgNoFixed=on  tSample=Task_L10ms  modeCode=Parameterless  modeRound=Zero
  Send CAN Message 2 : SF_CanService_Libs/Send CAN Message   typeCAN=Connected  channel=CAN_D  mEn=off  msgInfo=LeoDrive_vw_GOLF  msgItermStore=VehicleSignalStatus  msgIterm=VehicleSignalStatus  motoBit=off  flgNoFixed=on  tSample=Task_L10ms  modeCode=Parameterless  modeRound=Zero
  Send CAN Message 3 : SF_CanService_Libs/Send CAN Message   typeCAN=Connected  channel=CAN_D  mEn=off  msgInfo=LeoDrive_vw_GOLF  msgItermStore=VehicleDynamicsInfo  msgIterm=VehicleDynamicsInfo  motoBit=off  flgNoFixed=on  tSample=Task_L10ms  modeCode=Parameterless  modeRound=Zero
  Send CAN Message 4 : SF_CanService_Libs/Send CAN Message   typeCAN=Connected  channel=CAN_D  mEn=off  msgInfo=LeoDrive_vw_GOLF  msgItermStore=VehicleErrors  msgIterm=VehicleErrors  motoBit=off  flgNoFixed=on  tSample=Task_L10ms  modeCode=Parameterless  modeRound=Zero
  Steering Map reverse : Subsystem
  VehicleSpeed : Subsystem
  wires:
  In1/1 -> Bus Selector6/1, Bus Selector2/1, VehicleSpeed/1(In1), Bus Selector5/1, Bus Selector3/1, Bus Selector1/1, Bus Selector4/1, Bus Selector/1
  Bus Selector/1 -> "Send CAN Message "/2  "<GOLF_MotorRPM>"
  Bus Selector/2 -> "Send CAN Message "/3  "<GOLF_KL75>"
  Constant/1 -> "Send CAN Message "/1
  Bus Selector1/1 -> Send CAN Message 1/6  "<GOLF_AcceleratorRawValur>"
  Bus Selector1/2 -> Send CAN Message 1/7  "<GOLF_BrakePedalPos>"
  Bus Selector1/3 -> Send CAN Message 1/8  "<Steering_Angle>"
  Bus Selector2/7 -> Send CAN Message 2/7  "<GOLF_HandBrakeStatus>"
  Bus Selector2/6 -> Send CAN Message 2/6  "<mode>"
  Bus Selector2/5 -> Send CAN Message 2/5  "<GOLF_CurrentGear>"
  Bus Selector2/4 -> Send CAN Message 2/3  "<GOLF_HighBeam>"
  Chart/1(output) -> Send CAN Message 2/2
  Bus Selector2/1 -> Chart/1(left)  "<GOLF_BlinkerLeft>"
  Bus Selector2/2 -> Chart/2(right)  "<GOLF_BlinkerRight>"
  Bus Selector3/1 -> Steering Map reverse/1(Steering Wheel degree)  "<Steering_Angle>"
  VehicleSpeed/1(m/s) -> Send CAN Message 3/1
  Bus Selector6/1 -> Send CAN Message 2/1  "<GOLF_Fuel>"
  Constant5/1 -> Send CAN Message 2/8
  Constant6/1 -> Send CAN Message 2/4
  Bus Selector4/1 -> Send CAN Message 1/1  "<EPAS_DriverIntervention_overrideOvrMsr>"
  Bus Selector4/2 -> Send CAN Message 1/2  "<BBW_DriverIntervention>"
  Bus Selector4/3 -> Send CAN Message 1/3  "<GasPedalintervention>"
  Constant1/1 -> Send CAN Message 1/4
  Constant2/1 -> Send CAN Message 1/5
  Bus Selector5/1 -> Send CAN Message 4/1  "<isMotorRunning>"
  Bus Selector5/2 -> Send CAN Message 4/2  "<Kl75>"
  Bus Selector5/3 -> Send CAN Message 4/3  "<PDS_HeartbeatErr>"
  Bus Selector5/4 -> Send CAN Message 4/4  "<PDS_BUSErr>"
  Bus Selector5/5 -> Send CAN Message 4/5  "<By-wirePowerErr>"
  Bus Selector5/6 -> Send CAN Message 4/6  "<EPASPowerErr>"
  Bus Selector5/7 -> Send CAN Message 4/7  "<BrakePowerErr>"
  Bus Selector5/8 -> Send CAN Message 4/8  "<Throttle_ECU_HeartbeatErr>"
  Bus Selector5/9 -> Send CAN Message 4/10  "<EPAS_SystemErr>"
  Bus Selector5/10 -> Send CAN Message 4/11  "<EPAS_HeartbeatErr>"
  Bus Selector5/11 -> Send CAN Message 4/12  "<Brake_SystemErr>"
  Bus Selector5/12 -> Send CAN Message 4/13  "<Brake_HeartBeatErr>"
  Bus Selector5/13 -> Send CAN Message 4/14  "<PC_HeartBeatErr>"
  Constant3/1 -> Send CAN Message 4/9
  Bus Selector2/3 -> Chart/3(Hazard)  "<GOLF_HazardLight>"
  Steering Map reverse/1(Wheel Rad) -> Send CAN Message 3/2

== system Ecotron/Subsystem4/PDS ==
  In1 : Inport
  Bus Selector : BusSelector  OutputSignals=PDSscript.Msgtrigger,PDSscript.Channel,PDSscript.Onoff
  Subsystem : Subsystem
  wires:
  In1/1 -> Bus Selector/1
  Bus Selector/1 -> Subsystem/Trigger  "<Msgtrigger>"
  Bus Selector/2 -> Subsystem/1(Channel)  "<Channel>"
  Bus Selector/3 -> Subsystem/2(request)  "<Onoff>"

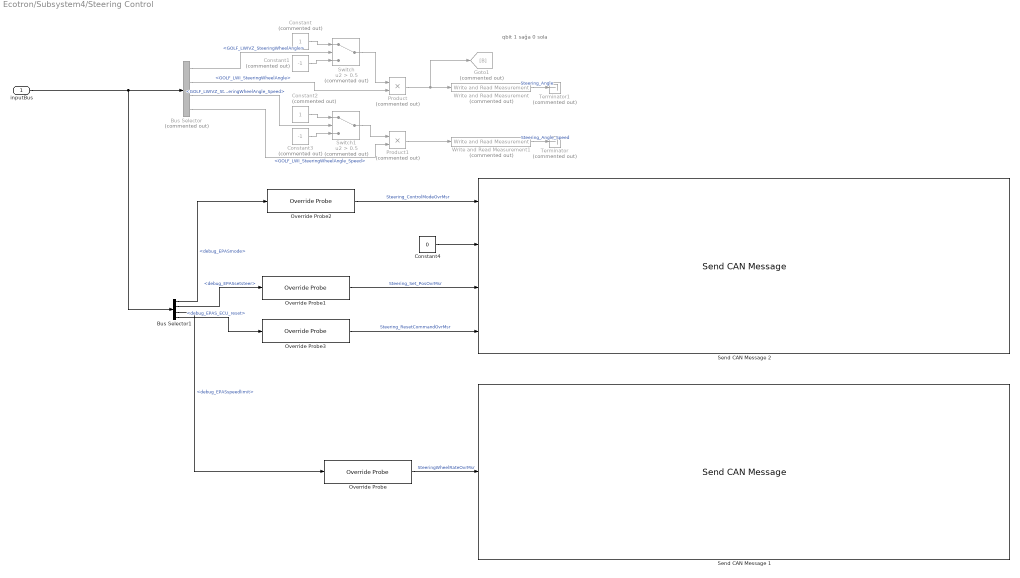
== system Ecotron/Subsystem4/Steering Control  ==
  note: qbit 1 sağa 0 sola
  inputBus : Inport
  " Override Probe" : CoderSF_BSW_Libs/Calibration & Measurement/ Override Probe  variableName=SteeringWheelRate  variableValue=0  overrideValue=0  variableDataType=single  variableMin=[]  variableMax=[]  variableUnitStr=""  variableDescStr=""
      settings: SourceProductName=EcoCoder Blocks
  " Override Probe1" : CoderSF_BSW_Libs/Calibration & Measurement/ Override Probe  variableName=Steering_Set_Pos  variableValue=0  overrideValue=0  variableDataType=single  variableMin=[]  variableMax=[]  variableUnitStr=""  variableDescStr=""
      settings: SourceProductName=EcoCoder Blocks
  " Override Probe2" : CoderSF_BSW_Libs/Calibration & Measurement/ Override Probe  variableName=Steering_ControlMode  variableValue=0  overrideValue=0  variableDataType=single  variableMin=[]  variableMax=[]  variableUnitStr=""  variableDescStr=""
      settings: SourceProductName=EcoCoder Blocks
  " Override Probe3" : CoderSF_BSW_Libs/Calibration & Measurement/ Override Probe  variableName=Steering_ResetCommand  variableValue=0  overrideValue=0  variableDataType=single  variableMin=[]  variableMax=[]  variableUnitStr=""  variableDescStr=""
      settings: SourceProductName=EcoCoder Blocks
  Bus Selector : BusSelector  Commented=on  OutputSignals=input.vehicle.LWI.GOLF_LWIVZ_SteeringWheelAngle,input.vehicle.LWI.GOLF_LWI_SteeringWheelAngle,input.vehicle.LWI.GOLF_LWIVZ_SteeringWheelAngle_Speed,input.vehicle.LWI.GOLF_LWI_SteeringWheelAngle_Speed
  Bus Selector1 : BusSelector  OutputSignals=debug_EPASmode,debug_EPASsetsteer,debug_EPASspeedlimit,debug_EPAS_ECU_reset
  Constant : Constant  Commented=on
  Constant1 : Constant  Commented=on  Value=-1
  Constant2 : Constant  Commented=on
  Constant3 : Constant  Commented=on  Value=-1
  Constant4 : Constant  Value=0
  Goto1 : Goto  Commented=on  GotoTag=B
  Product : Product  Commented=on
  Product1 : Product  Commented=on
  Send CAN Message 1 : SF_CanService_Libs/Send CAN Message   typeCAN=Connected  channel=CAN_C  mEn=off  msgInfo=RBF_DBW40_speedlimit  msgItermStore=Max_Speed_ID  msgIterm=Max_Speed_ID  motoBit=off  flgNoFixed=on  tSample=Task_L10ms  modeCode=Parameterless  modeRound=Zero
  Send CAN Message 2 : SF_CanService_Libs/Send CAN Message   typeCAN=Connected  channel=CAN_C  mEn=off  msgInfo=RBF_DBW40  msgItermStore=CommandMessage  msgIterm=CommandMessage  motoBit=off  flgNoFixed=on  tSample=Task_L10ms  modeCode=Parameterless  modeRound=Zero
  Switch : Switch  Commented=on  Criteria=u2 > Threshold  Threshold=0.5  OutDataTypeStr=single
  Switch1 : Switch  Commented=on  Criteria=u2 > Threshold  Threshold=0.5  OutDataTypeStr=single
  Terminator : Terminator  Commented=on
  Terminator1 : Terminator  Commented=on
  Write and Read Measurement : CoderSF_BSW_Libs/Calibration & Measurement/Write and Read Measurement  Commented=on  variable_name=Steering_Angle  variable_value=0  variable_type=single  numD=1  unitStr=""  descStr=""
      settings: AttributesFormatString=type:%<variable_type> Dimensions:%<numD>  SourceProductName=EcoCoder Blocks
  Write and Read Measurement1 : CoderSF_BSW_Libs/Calibration & Measurement/Write and Read Measurement  Commented=on  variable_name=Steering_Angle_Speed  variable_value=0  variable_type=single  numD=1  unitStr=""  descStr=""
      settings: AttributesFormatString=type:%<variable_type> Dimensions:%<numD>  SourceProductName=EcoCoder Blocks
  wires:
  " Override Probe3"/1 -> Send CAN Message 2/4  "Steering_ResetCommandOvrMsr"
  inputBus/1 -> Bus Selector1/1, Bus Selector/1
  Bus Selector/1 -> Switch/2  "<GOLF_LWIVZ_SteeringWheelAngle>"
  Bus Selector/2 -> Product/2  "<GOLF_LWI_SteeringWheelAngle>"
  Constant/1 -> Switch/1
  Constant1/1 -> Switch/3
  Switch/1 -> Product/1
  Product/1 -> Goto1/1, Write and Read Measurement/1
  Bus Selector/3 -> Switch1/2  "<GOLF_LWIVZ_SteeringWheelAngle_Speed>"
  Bus Selector/4 -> Product1/2  "<GOLF_LWI_SteeringWheelAngle_Speed>"
  Constant3/1 -> Switch1/3
  Constant2/1 -> Switch1/1
  Switch1/1 -> Product1/1
  Product1/1 -> Write and Read Measurement1/1
  " Override Probe"/1 -> Send CAN Message 1/1  "SteeringWheelRateOvrMsr"
  Write and Read Measurement1/1 -> Terminator/1  "Steering_Angle_Speed"
  Write and Read Measurement/1 -> Terminator1/1  "Steering_Angle"
  " Override Probe1"/1 -> Send CAN Message 2/3  "Steering_Set_PosOvrMsr"
  Constant4/1 -> Send CAN Message 2/2
  " Override Probe2"/1 -> Send CAN Message 2/1  "Steering_ControlModeOvrMsr"
  Bus Selector1/3 -> " Override Probe"/1  "<debug_EPASspeedlimit>"
  Bus Selector1/1 -> " Override Probe2"/1  "<debug_EPASmode>"
  Bus Selector1/2 -> " Override Probe1"/1  "<debug_EPASsetsteer>"
  Bus Selector1/4 -> " Override Probe3"/1  "<debug_EPAS_ECU_reset>"

== system Ecotron/Input/By-wire/PDS ==
  Bus Creator13 : BusCreator  Inputs=6
  Subsystem : Subsystem
  Subsystem1 : Subsystem
  Subsystem2 : Subsystem
  Subsystem3 : Subsystem
  Subsystem4 : Subsystem
  Subsystem6 : Subsystem
  PDS : Outport
  wires:
  Subsystem/1(Status) -> Bus Creator13/1
  Subsystem4/1(Status2) -> Bus Creator13/2
  Subsystem3/1(Current1) -> Bus Creator13/3
  Subsystem2/1(Current2) -> Bus Creator13/4
  Subsystem1/1(Current3) -> Bus Creator13/5
  Subsystem6/1(UnitedChannels) -> Bus Creator13/6
  Bus Creator13/1 -> PDS/1

== system Ecotron/Input/By-wire/Robeff Brake ECU ==
  Bus Creator : BusCreator  Inputs=3
  Robeff Brake FbMsg1 : Subsystem
  Robeff Brake FbMsg2 : Subsystem
  Robeff Brake FbMsg3 : Subsystem
  RBF_Brake : Outport
  wires:
  Robeff Brake FbMsg3/1("Msg3 ") -> Bus Creator/3  "EPAS_Msg3"
  Robeff Brake FbMsg2/1(Msg2) -> Bus Creator/2  "EPAS_Msg2"
  Bus Creator/1 -> RBF_Brake/1
  Robeff Brake FbMsg1/1(Msg1) -> Bus Creator/1  "EPAS_Msg1"

== system Ecotron/Input/By-wire/Robeff EPAS ECU ==
  Bus Creator : BusCreator  Inputs=3
  Robeff EPAS FbMsg1 : Subsystem
  Robeff EPAS FbMsg2 : Subsystem
  Robeff EPAS FbMsg3 : Subsystem
  EPAS : Outport
  wires:
  Robeff EPAS FbMsg1/1(Msg1) -> Bus Creator/1  "EPAS_Msg1"
  Bus Creator/1 -> EPAS/1
  Robeff EPAS FbMsg2/1(Msg2) -> Bus Creator/2  "EPAS_Msg2"
  Robeff EPAS FbMsg3/1("Msg3 ") -> Bus Creator/3  "EPAS_Msg3"
